simulink model "Inciso1D"  (R2023a)
settings: Solver=VariableStepAuto  StartTime=0.0  StopTime=250.0  RelTol=1e-3
settings Model: Creator=Daniela  LastModifiedBy=Daniela

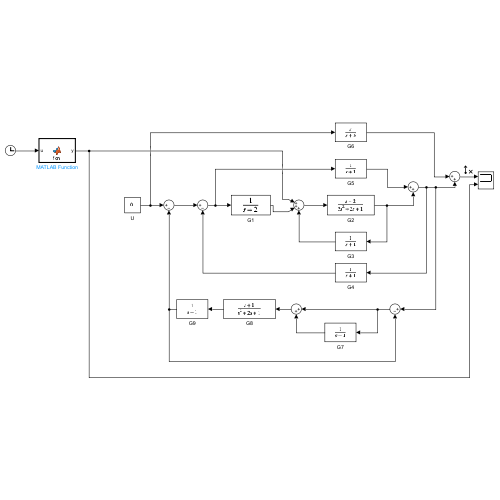
[thumbnail: Simulink's stored preview of the top-level diagram]
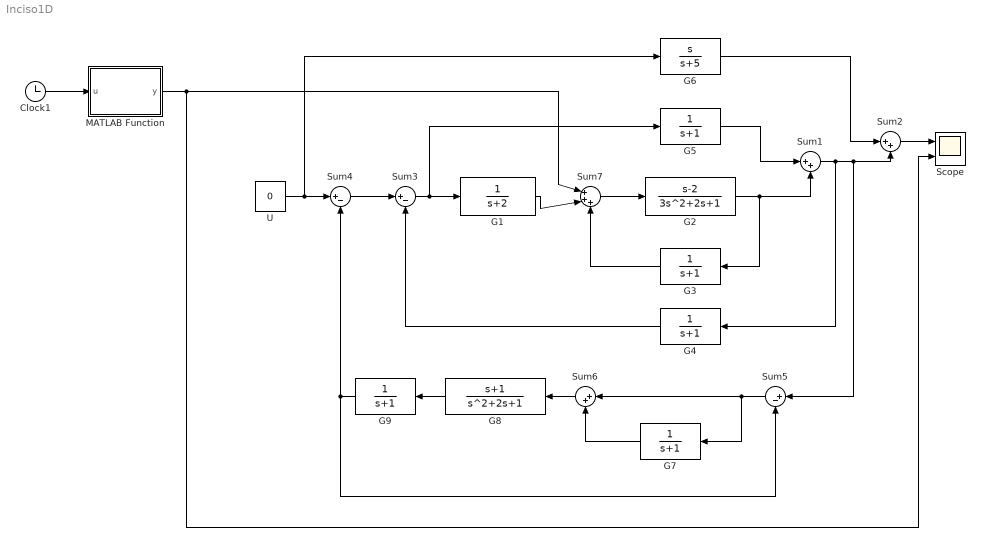
== system Inciso1D ==
  Clock1 : Clock
  G1 : TransferFcn  Numerator=[1 ]  Denominator=[1 2]
  G2 : TransferFcn  Numerator=[1 -2]  Denominator=[3 2 1]
  G{3..5,7,9} (5 alike) : TransferFcn  Denominator=[1 1]
  G6 : TransferFcn  Numerator=[1 0]  Denominator=[1 5]
  G8 : TransferFcn  Numerator=[1 1]
  MATLAB Function : MATLAB Function  TreatAsAtomicUnit=on
  Scope : Scope  NumInputPorts=2
  Sum1 : Sum  Inputs=|++
  Sum2 : Sum  Inputs=|++
  Sum3 : Sum  Inputs=|+-
  Sum4 : Sum  Inputs=|+-
  Sum5 : Sum  Inputs=|+-
  Sum6 : Sum  Inputs=|++
  Sum7 : Sum  Inputs=|+++
  U : Constant  Value=0
  wires:
  G1/1 -> Sum7/2
  G2/1 -> G3/1, Sum1/2
  Sum3/1 -> G5/1, G1/1
  G5/1 -> Sum1/1
  Sum4/1 -> Sum3/1
  G6/1 -> Sum2/1
  Sum1/1 -> G4/1, Sum5/1, Sum2/2
  Sum2/1 -> Scope/1
  G4/1 -> Sum3/2
  G8/1 -> G9/1
  Sum6/1 -> G8/1
  Sum5/1 -> G7/1, Sum6/1
  G7/1 -> Sum6/2
  G9/1 -> Sum4/2, Sum5/2
  Sum7/1 -> G2/1
  G3/1 -> Sum7/3
  Clock1/1 -> MATLAB Function/1(u)
  MATLAB Function/1(y) -> Scope/2, Sum7/1
  U/1 -> G6/1, Sum4/1

== matlab function Inciso1D/MATLAB Function ==
  data: u input; y output
function y = fcn(u)
y = exp(-0.1*u)*sin(0.2*pi*u);
